simulink model "bf_ranger_indi_continu"  (R2021a)
settings: Solver=VariableStepAuto  StartTime=0.0  StopTime=5  RelTol=1e-3
values from neighbouring files (symbols this model uses):
  Ah3 = blkdiag(Ah3, Ahc)    [ranger_sim.m]
  Ah7 = blkdiag(Ah7, Ahc)    [ranger_sim.m]
  Amc = d2c(Amd,'tustin')    [ranger_sim.m]
  Asc = d2c(Asd,'tustin')    [ranger_sim.m]
  Bh3 = blkdiag(Bh3, Bhc)    [ranger_sim.m]
  Bh7 = blkdiag(Bh7, Bhc)    [ranger_sim.m]
  Ch3 = blkdiag(Ch3, Chc)    [ranger_sim.m]
  Ch7 = blkdiag(Ch7, Chc)    [ranger_sim.m]
  Dh3 = blkdiag(Dh3, Dhc)    [ranger_sim.m]
  Dh7 = blkdiag(Dh7, Dhc)    [ranger_sim.m]
  G = [-10.67  10.67  0     0     0     0 0 ... (first row only)    [ranger_sim.m]
  G_inv = pinv(G)    [ranger_sim.m]
  G_thrust = [0 0 0 0 0 0 0 ... (first row only)    [ranger_sim.m]
  Kd = [10; 18; 18]    [ranger_sim.m]
  Kp = [4.1089; 4.7304; 7.36]    [ranger_sim.m]
settings Model: Creator=AutomZ2-RG02B04  LastModifiedBy=AutomZ2-RG02A02
settings SolverCC: AlgebraicLoopSolver=TrustRegion

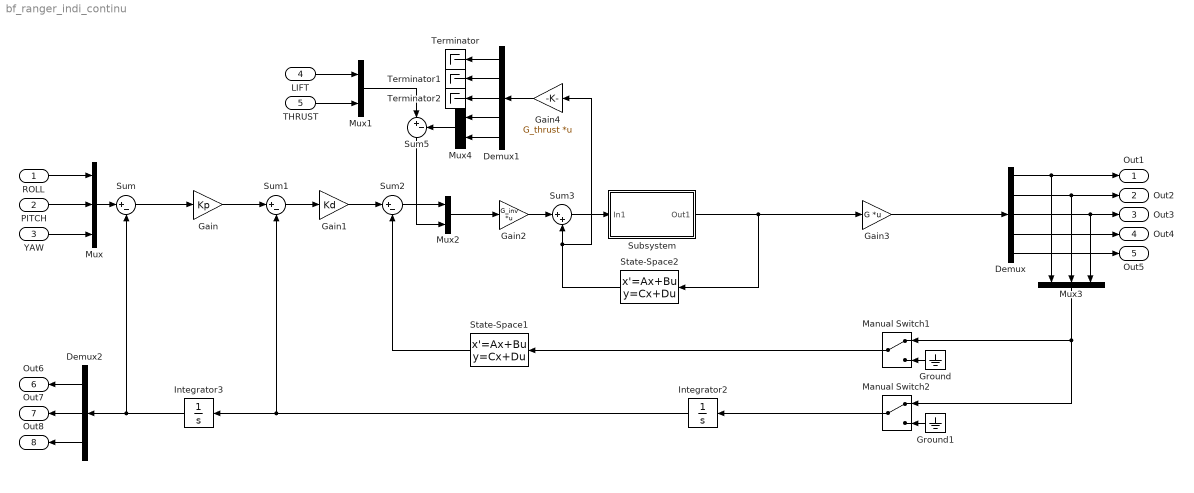
== system bf_ranger_indi_continu ==
  ROLL : Inport
  PITCH : Inport  Port=2
  YAW : Inport  Port=3
  LIFT : Inport  Port=4
  THRUST : Inport  Port=5
  Demux : Demux  Outputs=5
  Demux1 : Demux  Outputs=5
  Demux2 : Demux  Outputs=3
  Gain : Gain  Gain=Kp
  Gain1 : Gain  Gain=Kd
  Gain2 : Gain  Gain=G_inv  Multiplication=Matrix(K*u)
  Gain3 : Gain  Gain=G  Multiplication=Matrix(K*u)
  Gain4 : Gain  Gain=G_thrust  Multiplication=Matrix(K*u)
  Ground : Ground
  Ground1 : Ground
  Integrator2 : Integrator
  Integrator3 : Integrator
  Manual Switch1 : ManualSwitch
  Manual Switch2 : ManualSwitch
  Mux : Mux  Inputs=3
  Mux1 : Mux  Inputs=2
  Mux2 : Mux  Inputs=[3 2]
  Mux3 : Mux  Inputs=3
  Mux4 : Mux  Inputs=2
  State-Space1 : StateSpace  A=Ah3  B=Bh3  C=Ch3  D=Dh3  InitialCondition=0
  State-Space2 : StateSpace  A=Ah7  B=Bh7  C=Ch7  D=Dh7  InitialCondition=0
  Subsystem : Subsystem
  Sum{,1..2,5} (4 alike) : Sum  Inputs=|+-
  Sum3 : Sum  Inputs=|++
  Terminator : Terminator
  Terminator1 : Terminator
  Terminator2 : Terminator
  Out1 : Outport
  Out2 : Outport  Port=2
  Out3 : Outport  Port=3
  Out4 : Outport  Port=4
  Out5 : Outport  Port=5
  Out6 : Outport  Port=6
  Out7 : Outport  Port=7
  Out8 : Outport  Port=8
  wires:
  Sum/1 -> Gain/1
  Gain/1 -> Sum1/1
  Sum1/1 -> Gain1/1
  Gain1/1 -> Sum2/1
  Sum2/1 -> Mux2/1
  Gain2/1 -> Sum3/1
  Mux2/1 -> Gain2/1
  Sum3/1 -> Subsystem/1(In1)
  PITCH/1 -> Mux/2
  YAW/1 -> Mux/3
  Mux/1 -> Sum/1
  LIFT/1 -> Mux1/1
  THRUST/1 -> Mux1/2
  Demux/1 -> Mux3/1, Out1/1
  Demux/2 -> Mux3/2, Out2/1
  Demux/3 -> Out3/1, Mux3/3
  Demux/4 -> Out4/1
  Demux/5 -> Out5/1
  ROLL/1 -> Mux/1
  Gain3/1 -> Demux/1
  Integrator2/1 -> Sum1/2, Integrator3/1
  State-Space1/1 -> Sum2/2
  Subsystem/1(Out1) -> State-Space2/1, Gain3/1
  Integrator3/1 -> Sum/2, Demux2/1
  Demux2/1 -> Out6/1
  Demux2/2 -> Out7/1
  Demux2/3 -> Out8/1
  State-Space2/1 -> Gain4/1, Sum3/2
  Mux1/1 -> Sum5/1
  Sum5/1 -> Mux2/2
  Mux3/1 -> Manual Switch2/1, Manual Switch1/1
  Ground/1 -> Manual Switch1/2
  Manual Switch1/1 -> State-Space1/1
  Ground1/1 -> Manual Switch2/2
  Manual Switch2/1 -> Integrator2/1
  Demux1/3 -> Terminator2/1
  Demux1/4 -> Mux4/1
  Demux1/2 -> Terminator1/1
  Gain4/1 -> Demux1/1
  Mux4/1 -> Sum5/2
  Demux1/5 -> Mux4/2
  Demux1/1 -> Terminator/1

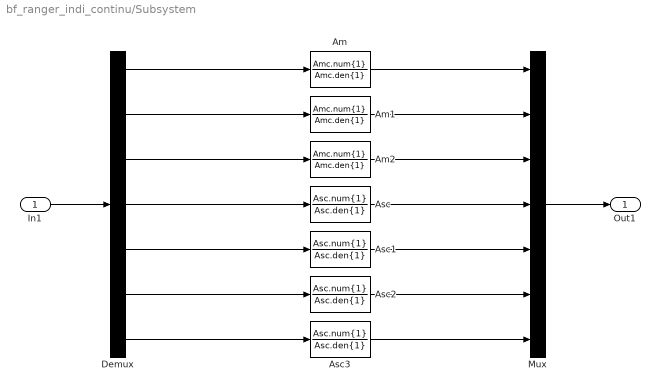
== system bf_ranger_indi_continu/Subsystem ==
  In1 : Inport
  Am : TransferFcn  Numerator=Amc.num{1}  Denominator=Amc.den{1}
  Am1 : TransferFcn  Numerator=Amc.num{1}  Denominator=Amc.den{1}
  Am2 : TransferFcn  Numerator=Amc.num{1}  Denominator=Amc.den{1}
  Asc{,1..3} (4 alike) : TransferFcn  Numerator=Asc.num{1}  Denominator=Asc.den{1}
  Demux : Demux  Outputs=7
  Mux : Mux  Inputs=7
  Out1 : Outport
  wires:
  Demux/5 -> Asc1/1
  Asc/1 -> Mux/4
  Demux/4 -> Asc/1
  Asc1/1 -> Mux/5
  Asc2/1 -> Mux/6
  Demux/6 -> Asc2/1
  Asc3/1 -> Mux/7
  Demux/7 -> Asc3/1
  In1/1 -> Demux/1
  Mux/1 -> Out1/1
  Demux/1 -> Am/1
  Am/1 -> Mux/1
  Am1/1 -> Mux/2
  Demux/2 -> Am1/1
  Am2/1 -> Mux/3
  Demux/3 -> Am2/1
